simulink model "LQR_control"  (R2023b)
settings: Solver=VariableStepAuto  StartTime=0.0  StopTime=20  RelTol=1e-3
undefined symbols (not defined in the file): g, K, k_d, k_energy, k_p, l, linear_limit, m, tau, X, Y, Z
libraries: sm_lib x12, nesl_utility x7, simulink_extras x2, fl_lib x1
settings Model: Creator=birad  LastModifiedBy=birad

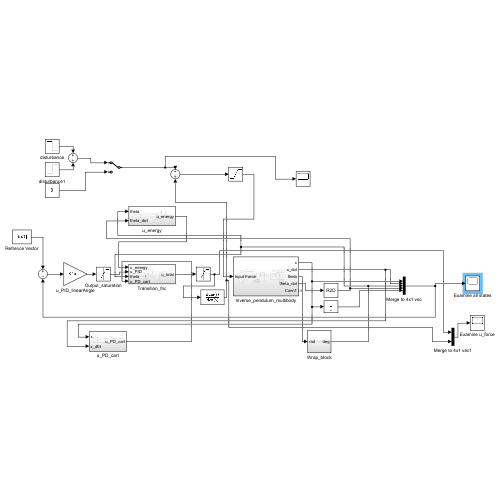
[thumbnail: Simulink's stored preview of the top-level diagram]
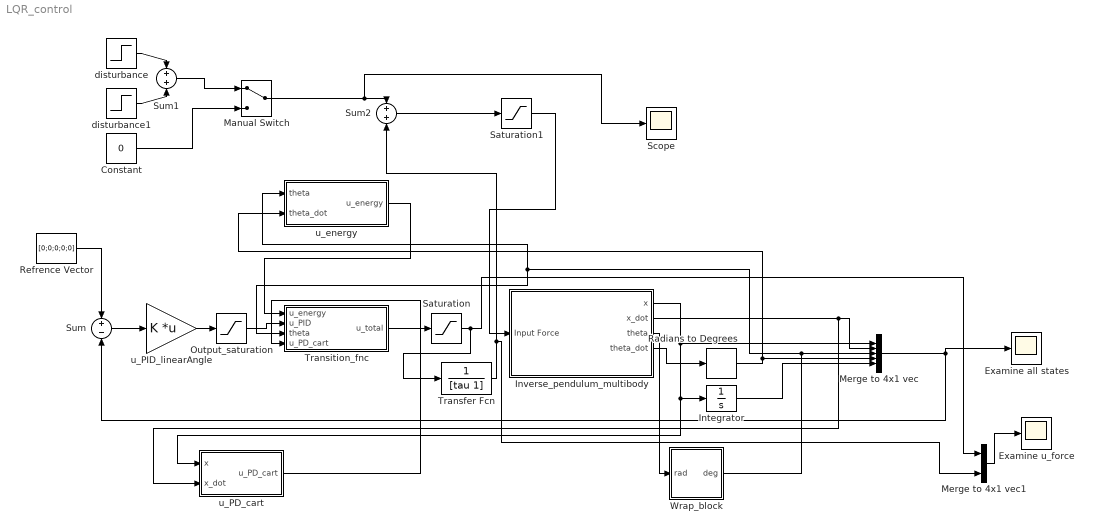
== system LQR_control ==
  Constant : Constant  Value=0
  Examine all states : Scope
  Examine u_force : Scope
  Integrator : Integrator
  Inverse_pendulum_multibody : Subsystem
  Manual Switch : ManualSwitch
  Merge to 4x1 vec : Mux  Inputs=5
  Merge to 4x1 vec1 : Mux  Inputs=2
  Output_saturation : Saturate  UpperLimit=300  LowerLimit=-300
  Radians to Degrees : simulink_extras/Transformations/Radians to Degrees
  Refrence Vector : Constant  Value=[0;0;0;0;0]  VectorParams1D=off
  Saturation : Saturate  UpperLimit=300  LowerLimit=-300
  Saturation1 : Saturate  UpperLimit=300  LowerLimit=-300
  Scope : Scope
  Sum : Sum  Inputs=+-
  Sum1 : Sum
  Sum2 : Sum
  Transfer Fcn : TransferFcn  Denominator=[tau 1]
  Transition_fnc : Subsystem
  Wrap_block : Subsystem
  disturbance : Step  Time=10  After=-200  SampleTime=1
  disturbance1 : Step  Time=9  After=200  SampleTime=1
  u_PD_cart : Subsystem
  u_PID_linearAngle : Gain  Gain=K  Multiplication=Matrix(K*u)
  u_energy : Subsystem
  wires:
  Inverse_pendulum_multibody/1(x) -> Integrator/1, u_PD_cart/1(x), Merge to 4x1 vec/1
  Inverse_pendulum_multibody/2(x_dot) -> u_PD_cart/2(x_dot), Merge to 4x1 vec/2
  Merge to 4x1 vec/1 -> Examine all states/1, Sum/2
  Refrence Vector/1 -> Sum/1
  Sum/1 -> u_PID_linearAngle/1
  u_energy/1(u_energy) -> Transition_fnc/1(u_energy)
  Inverse_pendulum_multibody/3(theta) -> Wrap_block/1(rad)
  Wrap_block/1(deg) -> Transition_fnc/3(theta), u_energy/1(theta), Merge to 4x1 vec/3
  Inverse_pendulum_multibody/4(theta_dot) -> Radians to Degrees/1
  Radians to Degrees/1 -> u_energy/2(theta_dot), Merge to 4x1 vec/4
  u_PID_linearAngle/1 -> Output_saturation/1
  Output_saturation/1 -> Transition_fnc/2(u_PID)
  u_PD_cart/1(u_PD_cart) -> Transition_fnc/4(u_PD_cart)
  Constant/1 -> Manual Switch/2
  Manual Switch/1 -> Scope/1, Sum2/1
  Transition_fnc/1(u_total) -> Saturation/1
  Sum2/1 -> Saturation1/1
  Saturation/1 -> Merge to 4x1 vec1/1, Transfer Fcn/1
  Integrator/1 -> Merge to 4x1 vec/5
  Transfer Fcn/1 -> Sum2/2, Merge to 4x1 vec1/2
  Merge to 4x1 vec1/1 -> Examine u_force/1
  Saturation1/1 -> Inverse_pendulum_multibody/1(Input Force)
  Sum1/1 -> Manual Switch/1
  disturbance/1 -> Sum1/1
  disturbance1/1 -> Sum1/2

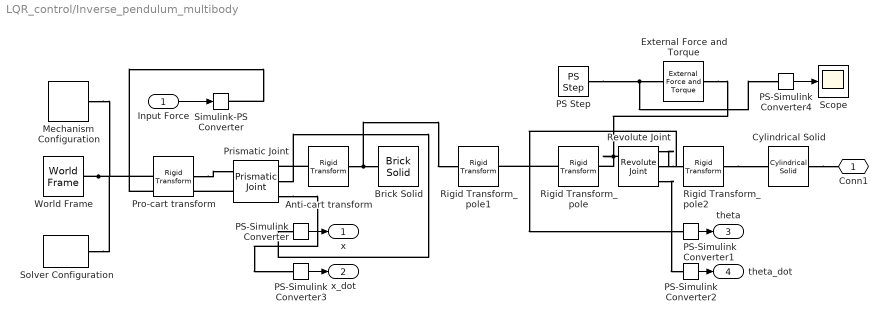
== system LQR_control/Inverse_pendulum_multibody ==
  Input Force : Inport
  Anti-cart transform : sm_lib/Frames and Transforms/Rigid Transform  TranslationMethod=None  TranslationStandardOffset=0  TranslationStandardOffsetUnits=m  TranslationStandardAxis=+Z  TranslationCartesianOffset=[0 0 0.5]  TranslationCartesianOffsetUnits=m  TranslationROffset=0  TranslationROffsetUnits=m  TranslationZOffset=0  TranslationZOffsetUnits=m  TranslationThetaOffset=0  TranslationThetaOffsetUnits=deg  RotationMethod=ArbitraryAxis  RotationAngleUnits=deg  RotationStandardAxis=+X  RotationAngle=90  RotationArbitraryAxis=[0 -1 0]  FollAlignAxisA=+X  BaseAlignAxisA=+Y  FollAlignAxisB=+Y  BaseAlignAxisB=+Z  RotationSequenceAxes=FollowerAxes  RotationSequence=XYX  RotationSequenceAngles=[0 0 0]  RotationSequenceAnglesUnits=deg  RotationMatrix=[1 0 0; 0 1 0; 0 0 1]  Quaternion=[1 0 0 0]
  Brick Solid : sm_lib/Body Elements/Brick Solid  GraphicAmbientColor=[0.15 0.15 0.15 1.0]  BasedOnType=Mass  BrickDimensions=[2 1 1]  BrickDimensionsUnits=m  CenterOfMass=[0 0 0]  CenterOfMassUnits=m  GraphicDiffuseColor=[0.5 0.5 0.5]  Density=1000  DensityUnits=kg/m^3  DoExposeReferenceFrame=on  GraphicEmissiveColor=[0.0 0.0 0.0 1.0]  ExportEntireGeometry=off  SerializedFrames=<Frames/>  MarkerShape=Sphere  MarkerSize=10  GraphicType=FromGeometry  InertiaType=CalculateFromGeometry  Mass=1  MassUnits=kg  MomentsOfInertia=[1 1 1]  MomentsOfInertiaUnits=kg*m^2  GraphicOpacity=1.0  ProductsOfInertia=[0 0 0]  ProductsOfInertiaUnits=kg*m^2  GraphicShininess=75  GraphicSpecularColor=[0.5 0.5 0.5 1.0]  GraphicVisPropType=SimpleVisualProperties
  Cylindrical Solid : sm_lib/Body Elements/Cylindrical Solid  GraphicAmbientColor=[0.15 0.15 0.15 1.0]  BasedOnType=Mass  CenterOfMass=[0 0 0]  CenterOfMassUnits=m  GraphicDiffuseColor=[0.5 0.5 0.5]  CylinderLength=3  CylinderLengthUnits=m  CylinderRadius=0.1  CylinderRadiusUnits=m  Density=1000  DensityUnits=kg/m^3  DoExposeReferenceFrame=on  GraphicEmissiveColor=[0.0 0.0 0.0 1.0]  ExportEntireGeometry=off  SerializedFrames=<Frames><Frame><Id>Frame1</Id><Value><Name>F1</Name><Origin><Source>GeometricFeature</Source><FeatureName>bottom surface</FeatureName></Origin><PrimaryAxis><DefinedDirection>+Z</DefinedDirection><Source>ReferenceFrame</Source><SourceDirection>+Z</SourceDirection><FeatureName></FeatureName></PrimaryAxis><SecondaryAxis><DefinedDirection>+X</DefinedDirection><Source>ReferenceFrame</Source><SourceDirection>+X</SourceDirection><FeatureName></FeatureName></SecondaryAxis></Value></Frame></Frames>  MarkerShape=Sphere  MarkerSize=10  GraphicType=FromGeometry  InertiaType=CalculateFromGeometry  Mass=1  MassUnits=kg  MomentsOfInertia=[1 1 1]  MomentsOfInertiaUnits=kg*m^2  GraphicOpacity=1.0  ProductsOfInertia=[0 0 0]  ProductsOfInertiaUnits=kg*m^2  GraphicShininess=75  GraphicSpecularColor=[0.5 0.5 0.5 1.0]  GraphicVisPropType=SimpleVisualProperties
  External Force and Torque : sm_lib/Forces and Torques/External Force and Torque  ForceResolutionFrame=AttachedFrame  EnableForceX=off  EnableForceY=off  EnableForceZ=off  EnableForce=off  TorqueResolutionFrame=AttachedFrame  EnableTorqueX=off  EnableTorqueY=off  EnableTorqueZ=on  EnableTorque=off
  Mechanism Configuration : sm_lib/Utilities/Mechanism Configuration  UniformGravity=Constant  GravityVector=[0 0 -9.80665]  GravityVectorUnits=m/s^2  LinearizationDelta=0.001  JointModeTransitionNonlinearIterations=2
  PS Step : fl_lib/Physical Signals/Sources/PS Step  step_time=9 s  initial_value=0  final_value=20
  PS-Simulink Converter{,1..4} (5 alike) : nesl_utility/PS-Simulink Converter  PhysicalDomain=network_engine_domain  SubClassName=ps_output  LeftPortType=input  RightPortType=output  PseudoPeriodic=off  Frequencies=[]  VectorFormat=inherit  Unit=inherit  AffineConversion=off
  Prismatic Joint : sm_lib/Joints/Prismatic Joint  JointMode=Normal  SenseConstraintForce=off  SenseConstraintForceX=off  SenseConstraintForceY=off  SenseConstraintForceZ=off  SenseConstraintTorque=off  SenseConstraintTorqueX=off  SenseConstraintTorqueY=off  SenseConstraintTorqueZ=off  SenseTotalForce=off  SenseTotalForceX=off  SenseTotalForceY=off  SenseTotalForceZ=off  SenseTotalTorque=off  SenseTotalTorqueX=off  SenseTotalTorqueY=off  SenseTotalTorqueZ=off  CompositeWrenchDir=FollowerOnBase  CompositeWrenchFrame=BaseFrame  EquilibriumPosition=0  EquilibriumPositionUnits=m  SpringStiffness=0  SpringStiffnessUnits=N/m  DampingCoefficient=0  DampingCoefficientUnits=N/(m/s)  TorqueActuationMode=InputTorque  MotionActuationMode=ComputedMotion  SensePosition=on  SenseVelocity=on  SenseAcceleration=off  SenseTorqueForce=off  SenseLowerLimitTorqueForce=off  SenseUpperLimitTorqueForce=off  LowerLimitSpecify=off  LowerLimitBound=-10  LowerLimitBoundUnits=m  LowerLimitStiffness=1e6  LowerLimitStiffnessUnits=N/m  LowerLimitDamping=1e3  LowerLimitDampingUnits=N/(m/s)  LowerLimitTransitionRegionWidth=1e-4  LowerLimitTransitionRegionWidthUnits=m  UpperLimitSpecify=off  UpperLimitBound=10  UpperLimitBoundUnits=m  UpperLimitStiffness=1e6  UpperLimitStiffnessUnits=N/m  UpperLimitDamping=1e3  UpperLimitDampingUnits=N/(m/s)  UpperLimitTransitionRegionWidth=1e-4  UpperLimitTransitionRegionWidthUnits=m  PositionTargetSpecify=on  PositionTargetPriority=High  PositionTargetValue=x_init  PositionTargetValueUnits=m  VelocityTargetSpecify=off  VelocityTargetPriority=High  VelocityTargetValue=0  VelocityTargetValueUnits=m/s
  Pro-cart transform : sm_lib/Frames and Transforms/Rigid Transform  TranslationMethod=None  TranslationStandardOffset=0  TranslationStandardOffsetUnits=m  TranslationStandardAxis=+Z  TranslationCartesianOffset=[0 0 0.5]  TranslationCartesianOffsetUnits=m  TranslationROffset=0  TranslationROffsetUnits=m  TranslationZOffset=0  TranslationZOffsetUnits=m  TranslationThetaOffset=0  TranslationThetaOffsetUnits=deg  RotationMethod=ArbitraryAxis  RotationAngleUnits=deg  RotationStandardAxis=+X  RotationAngle=90  RotationArbitraryAxis=[0 1 0]  FollAlignAxisA=+X  BaseAlignAxisA=+Y  FollAlignAxisB=+Y  BaseAlignAxisB=+Z  RotationSequenceAxes=FollowerAxes  RotationSequence=XYX  RotationSequenceAngles=[0 0 0]  RotationSequenceAnglesUnits=deg  RotationMatrix=[1 0 0; 0 1 0; 0 0 1]  Quaternion=[1 0 0 0]
  Revolute Joint : sm_lib/Joints/Revolute Joint  JointMode=Normal  SenseConstraintForce=off  SenseConstraintForceX=off  SenseConstraintForceY=off  SenseConstraintForceZ=off  SenseConstraintTorque=off  SenseConstraintTorqueX=off  SenseConstraintTorqueY=off  SenseConstraintTorqueZ=off  SenseTotalForce=off  SenseTotalForceX=off  SenseTotalForceY=off  SenseTotalForceZ=off  SenseTotalTorque=off  SenseTotalTorqueX=off  SenseTotalTorqueY=off  SenseTotalTorqueZ=off  CompositeWrenchDir=FollowerOnBase  CompositeWrenchFrame=BaseFrame  EquilibriumPosition=0  EquilibriumPositionUnits=deg  SpringStiffness=0  SpringStiffnessUnits=N*m/deg  DampingCoefficient=0  DampingCoefficientUnits=N*m/(deg/s)  TorqueActuationMode=InputTorque  MotionActuationMode=ComputedMotion  SensePosition=on  SenseVelocity=on  SenseAcceleration=off  SenseTorqueForce=off  SenseLowerLimitTorqueForce=off  SenseUpperLimitTorqueForce=off  LowerLimitSpecify=off  LowerLimitBound=-20  LowerLimitBoundUnits=deg  LowerLimitStiffness=1e4  LowerLimitStiffnessUnits=N*m/deg  LowerLimitDamping=10  LowerLimitDampingUnits=N*m/(deg/s)  LowerLimitTransitionRegionWidth=0.1  LowerLimitTransitionRegionWidthUnits=deg  UpperLimitSpecify=off  UpperLimitBound=20  UpperLimitBoundUnits=deg  UpperLimitStiffness=1e4  UpperLimitStiffnessUnits=N*m/deg  UpperLimitDamping=10  UpperLimitDampingUnits=N*m/(deg/s)  UpperLimitTransitionRegionWidth=0.1  UpperLimitTransitionRegionWidthUnits=deg  PositionTargetSpecify=on  PositionTargetPriority=High  PositionTargetValue=theta_init  PositionTargetValueUnits=rad  VelocityTargetSpecify=off  VelocityTargetPriority=High  VelocityTargetValue=1.05  VelocityTargetValueUnits=rad/s
  Rigid Transform_pole : sm_lib/Frames and Transforms/Rigid Transform  TranslationMethod=None  TranslationStandardOffset=0  TranslationStandardOffsetUnits=m  TranslationStandardAxis=+Z  TranslationCartesianOffset=[0 -0.5 0]  TranslationCartesianOffsetUnits=m  TranslationROffset=0  TranslationROffsetUnits=m  TranslationZOffset=0  TranslationZOffsetUnits=m  TranslationThetaOffset=0  TranslationThetaOffsetUnits=deg  RotationMethod=ArbitraryAxis  RotationAngleUnits=deg  RotationStandardAxis=+X  RotationAngle=90  RotationArbitraryAxis=[1 0 0]  FollAlignAxisA=+X  BaseAlignAxisA=+Y  FollAlignAxisB=+Y  BaseAlignAxisB=+Z  RotationSequenceAxes=FollowerAxes  RotationSequence=XYX  RotationSequenceAngles=[0 0 0]  RotationSequenceAnglesUnits=deg  RotationMatrix=[1 0 0; 0 1 0; 0 0 1]  Quaternion=[1 0 0 0]
  Rigid Transform_pole1 : sm_lib/Frames and Transforms/Rigid Transform  TranslationMethod=Cartesian  TranslationStandardOffset=0  TranslationStandardOffsetUnits=m  TranslationStandardAxis=+Z  TranslationCartesianOffset=[0 0 0.5]  TranslationCartesianOffsetUnits=m  TranslationROffset=0  TranslationROffsetUnits=m  TranslationZOffset=0  TranslationZOffsetUnits=m  TranslationThetaOffset=0  TranslationThetaOffsetUnits=deg  RotationMethod=None  RotationAngleUnits=deg  RotationStandardAxis=+X  RotationAngle=90  RotationArbitraryAxis=[1 0 0]  FollAlignAxisA=+X  BaseAlignAxisA=+Y  FollAlignAxisB=+Y  BaseAlignAxisB=+Z  RotationSequenceAxes=FollowerAxes  RotationSequence=XYX  RotationSequenceAngles=[0 0 0]  RotationSequenceAnglesUnits=deg  RotationMatrix=[1 0 0; 0 1 0; 0 0 1]  Quaternion=[1 0 0 0]
  Rigid Transform_pole2 : sm_lib/Frames and Transforms/Rigid Transform  TranslationMethod=None  TranslationStandardOffset=0  TranslationStandardOffsetUnits=m  TranslationStandardAxis=+Z  TranslationCartesianOffset=[0 0 0.5]  TranslationCartesianOffsetUnits=m  TranslationROffset=0  TranslationROffsetUnits=m  TranslationZOffset=0  TranslationZOffsetUnits=m  TranslationThetaOffset=0  TranslationThetaOffsetUnits=deg  RotationMethod=ArbitraryAxis  RotationAngleUnits=deg  RotationStandardAxis=+X  RotationAngle=-90  RotationArbitraryAxis=[1 0 0]  FollAlignAxisA=+X  BaseAlignAxisA=+Y  FollAlignAxisB=+Y  BaseAlignAxisB=+Z  RotationSequenceAxes=FollowerAxes  RotationSequence=XYX  RotationSequenceAngles=[0 0 0]  RotationSequenceAnglesUnits=deg  RotationMatrix=[1 0 0; 0 1 0; 0 0 1]  Quaternion=[1 0 0 0]
  Scope : Scope
  Simulink-PS Converter : nesl_utility/Simulink-PS Converter  PhysicalDomain=network_engine_domain  SubClassName=ps_input  LeftPortType=input  RightPortType=output  PseudoPeriodic=off  Frequencies=[]  NoiseDistribution=none  NoiseParameters=[]  Unit=1  AffineConversion=off  FilteringAndDerivatives=provide  SimscapeFilterOrder=1  InputFilterTimeConstant=0.001  UdotUserProvided=0
  Solver Configuration : nesl_utility/Solver Configuration  PhysicalDomain=network_engine_domain  SubClassName=solver  LeftPortType=input  RightPortType=generic  Tones=[]  Harmonics=[]  SimulateNoise=off  Profile=off  UseLocalSampling=off  EnableSwitchedLinearOptims=on  FrequencyDomain=off  UseCCode=off  RelTol=0.001  AbsTol=0.001  MinStep=1e-09  ToWorkspace=off  RevertToSquareIcSolve=off  NumHomotopyIterations=100  PhasorMode=off  PhasorModeNumHarmonics=1  ConsistencySolver=NEWTON_XTOL_AFTER_FTOL  IndexReductionMethod=DerivativeReplacement  DoDC=off  ResidualTolerance=1e-09  ConsistencyTolSource=GLOBAL  ConsistencyAbsTol=0.001  ConsistencyRelTol=0.001  ConsistencyTolFactor=0.001  UseLocalSolver=off  LocalSolverChoice=NE_BACKWARD_EULER_ADVANCER  ResolveIndetEquations=on  FunctionEvalNumThread=1  LocalSolverSampleTime=0.001  DoFixedCost=off  MaxNonlinIter=3  MaxModeIter=2  ComputeImpulses=off  ImpulseIterations=2  LinearAlgebra=auto  LinearAlgebraNumThread=0  EquationFormulation=NE_TIME_EF  DelaysMemoryBudget=1024  AutomaticFiltering=on  FilteringTimeConstant=0.001  PartitionStorageMethod=AS_NEEDED  PartitionMemoryBudget=1024  PartitionMethod=ROBUST  MultibodyUseLocalSolver=off  MultibodyLocalSolverChoice=ODE1  MultibodyLocalSolverSampleTime=0.001
  World Frame : sm_lib/Frames and Transforms/World Frame
  Conn1 : PMIOPort  Side=Right
  x : Outport
  x_dot : Outport  Port=2
  theta : Outport  Port=3
  theta_dot : Outport  Port=4
  wires:
  PS-Simulink Converter/1 -> x/1
  Input Force/1 -> Simulink-PS Converter/1
  PS-Simulink Converter1/1 -> theta/1
  PS-Simulink Converter3/1 -> x_dot/1
  PS-Simulink Converter2/1 -> theta_dot/1
  PS-Simulink Converter4/1 -> Scope/1
  connections:
  Revolute Joint/LConn1 -- Rigid Transform_pole/RConn1 -- External Force and Torque/RConn1
  Pro-cart transform/RConn1 -- Prismatic Joint/LConn1
  Anti-cart transform/LConn1 -- Prismatic Joint/RConn1
  World Frame/RConn1 -- Solver Configuration/RConn1 -- Pro-cart transform/LConn1 -- Mechanism Configuration/RConn1
  Anti-cart transform/RConn1 -- Rigid Transform_pole1/LConn1 -- Brick Solid/RConn1
  Rigid Transform_pole/LConn1 -- Rigid Transform_pole1/RConn1
  Rigid Transform_pole2/RConn1 -- Cylindrical Solid/LConn1
  Revolute Joint/RConn2 -- PS-Simulink Converter1/LConn1
  Revolute Joint/RConn1 -- Rigid Transform_pole2/LConn1
  Prismatic Joint/RConn2 -- PS-Simulink Converter/LConn1
  Cylindrical Solid/RConn1 -- Conn1/RConn1
  Revolute Joint/RConn3 -- PS-Simulink Converter2/LConn1
  Prismatic Joint/RConn3 -- PS-Simulink Converter3/LConn1
  Prismatic Joint/LConn2 -- Simulink-PS Converter/RConn1
  PS Step/RConn1 -- PS-Simulink Converter4/LConn1 -- External Force and Torque/LConn1

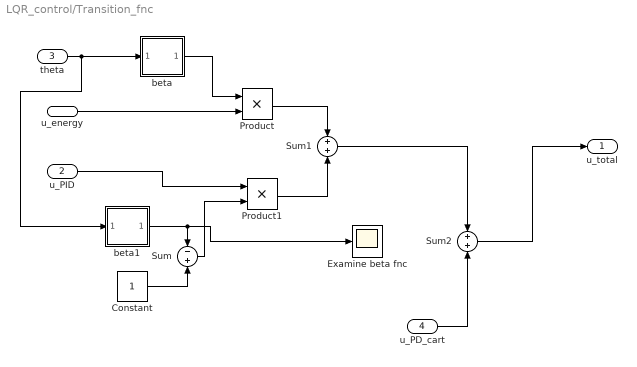
== system LQR_control/Transition_fnc ==
  u_energy : Inport
  u_PID : Inport  Port=2
  theta : Inport  Port=3
  u_PD_cart : Inport  Port=4
  Constant : Constant
  Examine beta fnc : Scope
  Product : Product
  Product1 : Product
  Sum : Sum  Inputs=-+
  Sum1 : Sum
  Sum2 : Sum
  beta : Subsystem
  beta1 : Subsystem
  u_total : Outport
  wires:
  theta/1 -> beta1/1(theta), beta/1(theta)
  u_energy/1 -> Product/2
  beta/1(Output) -> Product/1
  beta1/1(Output) -> Examine beta fnc/1, Sum/1
  Constant/1 -> Sum/2
  Sum/1 -> Product1/2
  u_PID/1 -> Product1/1
  Product/1 -> Sum1/1
  Product1/1 -> Sum1/2
  Sum1/1 -> Sum2/1
  u_PD_cart/1 -> Sum2/2
  Sum2/1 -> u_total/1

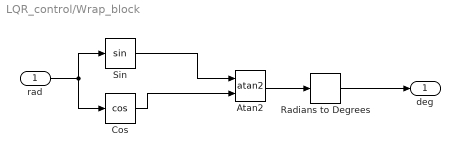
== system LQR_control/Wrap_block ==
  rad : Inport
  Atan2 : Trigonometry  Operator=atan2
  Cos : Trigonometry  Operator=cos
  Radians to Degrees : simulink_extras/Transformations/Radians to Degrees
  Sin : Trigonometry
  deg : Outport
  wires:
  rad/1 -> Sin/1, Cos/1
  Atan2/1 -> Radians to Degrees/1
  Radians to Degrees/1 -> deg/1
  Sin/1 -> Atan2/1
  Cos/1 -> Atan2/2

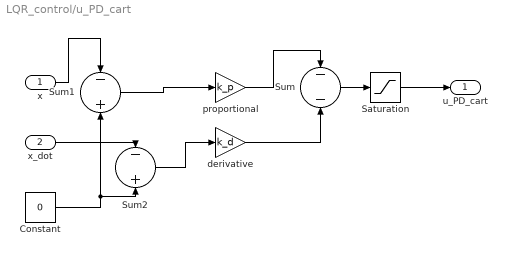
== system LQR_control/u_PD_cart ==
  x : Inport
  x_dot : Inport  Port=2
  Constant : Constant  Value=0
  Saturation : Saturate  UpperLimit=300  LowerLimit=-300
  Sum : Sum  Inputs=--
  Sum1 : Sum  Inputs=-+
  Sum2 : Sum  Inputs=-+
  derivative : Gain  Gain=k_d
  proportional : Gain  Gain=k_p
  u_PD_cart : Outport
  wires:
  proportional/1 -> Sum/1
  derivative/1 -> Sum/2
  x/1 -> Sum1/1
  Constant/1 -> Sum2/2, Sum1/2
  Sum1/1 -> proportional/1
  x_dot/1 -> Sum2/1
  Sum2/1 -> derivative/1
  Sum/1 -> Saturation/1
  Saturation/1 -> u_PD_cart/1

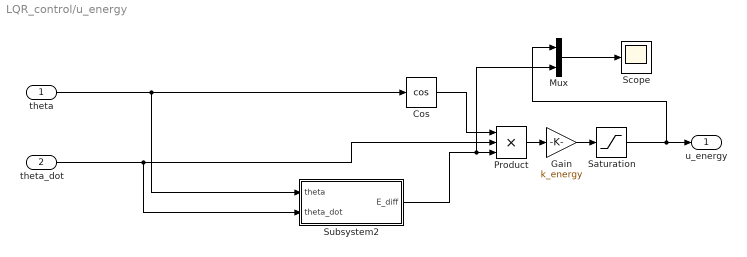
== system LQR_control/u_energy ==
  theta : Inport
  theta_dot : Inport  Port=2
  Cos : Trigonometry  Operator=cos
  Gain : Gain  Gain=k_energy
  Mux : Mux  Inputs=2
  Product : Product  Inputs=3
  Saturation : Saturate  UpperLimit=300  LowerLimit=-300
  Scope : Scope
  Subsystem2 : Subsystem
  u_energy : Outport
  wires:
  Product/1 -> Gain/1
  Gain/1 -> Saturation/1
  theta/1 -> Subsystem2/1(theta), Cos/1
  Cos/1 -> Product/1
  theta_dot/1 -> Subsystem2/2(theta_dot), Product/2
  Subsystem2/1(E_diff) -> Mux/2, Product/3
  Mux/1 -> Scope/1
  Saturation/1 -> Mux/1, u_energy/1

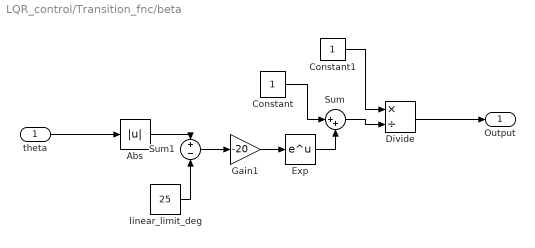
== system LQR_control/Transition_fnc/beta ==
  theta : Inport
  Abs : Abs  SaturateOnIntegerOverflow=off
  Constant : Constant
  Constant1 : Constant
  Divide : Product  Inputs=*/
  Exp : Math
  Gain1 : Gain  Gain=-20
  Sum : Sum  Inputs=|++
  Sum1 : Sum  Inputs=+-
  linear_limit_deg : Constant  Value=25
  Output : Outport
  wires:
  Divide/1 -> Output/1
  Exp/1 -> Sum/2
  Constant/1 -> Sum/1
  linear_limit_deg/1 -> Sum1/2
  Gain1/1 -> Exp/1
  Sum1/1 -> Gain1/1
  Abs/1 -> Sum1/1
  theta/1 -> Abs/1
  Constant1/1 -> Divide/1
  Sum/1 -> Divide/2

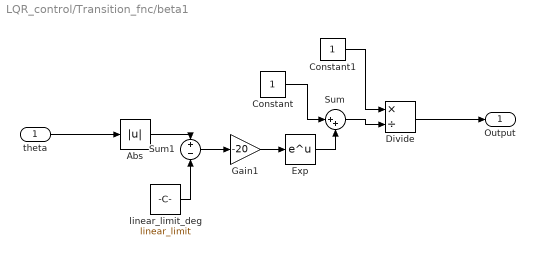
== system LQR_control/Transition_fnc/beta1 ==
  theta : Inport
  Abs : Abs  SaturateOnIntegerOverflow=off
  Constant : Constant
  Constant1 : Constant
  Divide : Product  Inputs=*/
  Exp : Math
  Gain1 : Gain  Gain=-20
  Sum : Sum  Inputs=|++
  Sum1 : Sum  Inputs=+-
  linear_limit_deg : Constant  Value=linear_limit
  Output : Outport
  wires:
  Sum/1 -> Divide/2
  Constant1/1 -> Divide/1
  theta/1 -> Abs/1
  Abs/1 -> Sum1/1
  Sum1/1 -> Gain1/1
  Gain1/1 -> Exp/1
  linear_limit_deg/1 -> Sum1/2
  Constant/1 -> Sum/1
  Exp/1 -> Sum/2
  Divide/1 -> Output/1

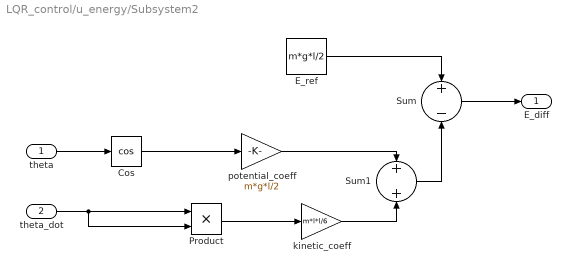
== system LQR_control/u_energy/Subsystem2 ==
  theta : Inport
  theta_dot : Inport  Port=2
  Cos : Trigonometry  Operator=cos
  E_ref : Constant  Value=m*g*l/2
  Product : Product
  Sum : Sum  Inputs=+-
  Sum1 : Sum
  kinetic_coeff : Gain  Gain=m*l*l/6
  potential_coeff : Gain  Gain=m*g*l/2
  E_diff : Outport
  wires:
  E_ref/1 -> Sum/1
  theta_dot/1 -> Product/2, Product/1
  Product/1 -> kinetic_coeff/1
  kinetic_coeff/1 -> Sum1/2
  potential_coeff/1 -> Sum1/1
  Sum1/1 -> Sum/2
  theta/1 -> Cos/1
  Cos/1 -> potential_coeff/1
  Sum/1 -> E_diff/1
